simulink model "r4_pfb_fir"  (Simulink 7.0)
settings: Solver=FixedStepDiscrete  SolverMode=SingleTasking  StartTime=0.0  StopTime=10.0  RelTol=1e-3
undefined symbols (not defined in the file): pfb_coefs
libraries: xbsIndex_r4 x385, xps_library x1
(part 13 of 27)

== system r4_pfb_fir/fir_1/fir_tap_2/fir_coef ==
  data_in : Inport  OutDataType=sfix(16)  OutScaling=2^0
  sum_in : Inport  Port=2  OutDataType=sfix(16)  OutScaling=2^0
  sync_in : Inport  Port=3  OutDataType=sfix(16)  OutScaling=2^0
  c_gen : Subsystem  mask(Coefficient Generator){coefs=[-0.000375660323525046;-0.00112528207646786;-0.00187263770065757;-0.00261772609063303;-0.00336054616203061;-0.00410109685156988;-0.00483937711704019;-0.00557538593728603;-0.00630912231219222;-0.00704058526266978;-0.00776977383064064;-0.00849668707902262;-0.00922132409171369;-0.00994368397357705;-0.0106637658504249;-0.0113815688690025;-0.0120970921969721;-0.0128103350228962;-0.0135212965562215;-0.0142299760272615;-0.0149363726871797;-0.0156404858079725;-0.0163423146824514;-0.0170418586242254;-0.0177391169676835;-0.0184340890679761;-0.0191267743009973;-0.0198171720633655;-0.0205052817724058;-0.0211911028661302;-0.0218746348032188;-0.0225558770630009;-0.0232348291454347;-0.0239114905710882;-0.0245858608811188;-0.0252579396372536;-0.0259277264217688;-0.0265952208374693;-0.0272604225076676;-0.0279233310761635;-0.0285839462072226;-0.0292422675855545;-0.0298982949162921;-0.0305520279249694;-0.0312034663574997;-0.031852609980153;-0.0324994585795345;-0.0331440119625613;-0.0337862699564402;-0.0344262324086442;-0.0350638991868898;-0.0356992701791137;-0.0363323452934489;-0.0369631244582015;-0.0375916076218262;-0.0382177947529027;-0.0388416858401109;-0.0394632808922069;-0.0400825799379981;-0.0406995830263182;-0.0413142902260021;-0.0419267016258609;-0.0425368173346564;-0.0431446374810749;-0.0437501622137022;-0.0443533917009969;-0.0449543261312647;-0.0455529657126312;-0.0461493106730163;-0.0467433612601067;-0.047335117741329;-0.0479245804038229;-0.0485117495544134;-0.0490966255195838;-0.0496792086454471;-0.0502594992977191;-0.0508374978616896;-0.0514132047421944;-0.0519866203635867;-0.0525577451697087;-0.0531265796238626;-0.0536931242087811;-0.0542573794265993;-0.0548193457988244;-0.0553790238663066;-0.0559364141892089;-0.0564915173469777;-0.0570443339383125;-0.0575948645811356;-0.0581431099125613;-0.058689070588866;-0.0592327472854569;-0.0597741406968409;-0.0603132515365938;-0.0608500805373288;-0.0613846284506648;-0.0619168960471949;-0.0624468841164546;-0.0629745934668896;-0.0635000249258237;-0.064023179339426;-0.0645440575726791;-0.0650626605093458;-0.0655789890519362;-0.0660930441216749;-0.0666048266584676;-0.0671143376208679;-0.067621577986043;-0.0681265487497408;-0.0686292509262558;-0.0691296855483946;-0.0696278536674418;-0.0701237563531258;-0.0706173946935843;-0.071108769795329;-0.071597882783211;-0.0720847348003859;-0.0725693270082785;-0.0730516605865468;-0.0735317367330474;-0.0740095566637989;-0.0744851216129466;-0.0749584328327259;-0.0754294915934268;-0.0758982991833568;-0.0763648569088048;-0.0768291660940042;-0.0772912280810962;-0.0777510442300928;-0.0782086159188393;-0.0786639445429775;-0.0791170315159078;-0.0795678782687517;-0.0800164862503141;-0.0804628569270452;-0.0809069917830028;-0.0813488923198131;-0.0817885600566336;-0.0822259965301136;-0.0826612032943558;-0.0830941819208773;-0.0835249339985711;-0.0839534611336661;-0.0843797649496887;-0.0848038470874227;-0.0852257092048699;-0.0856453529772106;-0.0860627800967632;-0.0864779922729447;-0.0868909912322302;-0.0873017787181127;-0.0877103564910625;-0.0881167263284868;-0.0885208900246886;-0.0889228493908263;-0.0893226062548723;-0.0897201624615717;-0.0901155198724016;-0.0905086803655288;-0.0908996458357691;-0.0912884181945446;-0.0916749993698427;-0.0920593913061736;-0.0924415959645284;-0.0928216153223364;-0.0931994513734234;-0.0935751061279683;-0.0939485816124612;-0.09431987986966;-0.0946890029585477;-0.0950559529542894;-0.0954207319481889;-0.0957833420476455;-0.0961437853761105;-0.0965020640730433;-0.0968581802938682;-0.0972121362099301;-0.0975639340084509;-0.0979135758924848;-0.0982610640808748;-0.0986064008082076;-0.0989495883247697;-0.0992906288965024;-0.0996295248049575;-0.0999662783472516;-0.100300891836022;-0.100633367599381;-0.100963707980872;-0.101291915339421;-0.101617992049296;-0.101941940500055;-0.102263763096507;-0.102583462258662;-0.102901040421687;-0.103216500035856;-0.103529843566511;-0.103841073494009;-0.104150192313679;-0.104457202535775;-0.104762106685429 ...(+16057 chars)], n_bits=9, bin_pt=8, log2_cpc=0, use_bram=on}
      mask prompts: coefs "Coefficients"; n_bits "Number of Bits"; bin_pt "Binary Point"; log2_cpc "Log2 Cycles per Coefficient"; use_bram "Use BRAM"
      mask help: A coefficient generator.
      settings: AttributesFormatString=|
      | 1024 coefs in bram
      | 9_8 out/1
      mask Help:
      | <pre>
      | Description::
      | 
      | A coefficient generator.
      | 
      | Mask Parameters::
      | 
      | Coefficiants (coefs): The coefficients to output.  These should be specified as doubles.
      | They will be rounded/saturated according to the specified number of bits (n_bits)
      | and binary point (bin_pt).
      | 
      | Number of Coefficient Bits (n_bits): The number of bits used for the fixed point binary
      | representation of the coefficients.
      | 
      | Coefficient Binary Point (bin_pt): The binary point of the fixed point binary representation
      | of the coefficients.
      | 
      | Log2 Cycles per Coefficient (log2_cpc): The log2 value of the number of cycles per coefficient.
      | Must be a non-negative integer (i.e. cycles per coefficient must be a power of 2).
      | 
      | Use BRAM (use_bram): Check this checkbox to store coefficients in BRAM.
      | If unchecked, the coefficients will be sored in distributed memory (i.e. slices).
      | </pre>
  data_delay : xbsIndex_r4/Delay  en=off  latency=1  dbl_ovrd=off  reg_retiming=off  block_type=delay
      settings: xl_area=[0, 0, 0, 0, 0, 0, 0]
  sum_delay : xbsIndex_r4/Delay  en=off  latency=1  dbl_ovrd=off  reg_retiming=off  block_type=delay
      settings: xl_area=[0, 0, 0, 0, 0, 0, 0]
  sync_delay : xbsIndex_r4/Delay  en=off  latency=1  dbl_ovrd=off  reg_retiming=off  block_type=delay
      settings: xl_area=[0, 0, 0, 0, 0, 0, 0]
  data_out : Outport  OutDataType=sfix(16)  OutScaling=2^0
  sum_out : Outport  Port=2  OutDataType=sfix(16)  OutScaling=2^0
  coef : Outport  Port=3  OutDataType=sfix(16)  OutScaling=2^0
  sync_out : Outport  Port=4  OutDataType=sfix(16)  OutScaling=2^0
  wires:
  c_gen/1(coef_out) -> coef/1
  sum_delay/1 -> sum_out/1
  sum_in/1 -> sum_delay/1
  sync_in/1 -> c_gen/1(sync_in), sync_delay/1
  sync_delay/1 -> sync_out/1
  data_delay/1 -> data_out/1
  data_in/1 -> data_delay/1

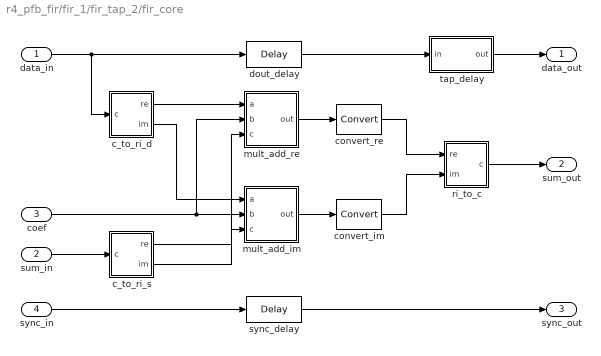
== system r4_pfb_fir/fir_1/fir_tap_2/fir_core ==
  data_in : Inport  OutDataType=sfix(16)  OutScaling=2^0
  sum_in : Inport  Port=2  OutDataType=sfix(16)  OutScaling=2^0
  coef : Inport  Port=3  OutDataType=sfix(16)  OutScaling=2^0
  sync_in : Inport  Port=4  OutDataType=sfix(16)  OutScaling=2^0
  c_to_ri_d : Subsystem  mask(Complex to Real-Imag){n_bits=8, bin_pt=7}
      mask prompts: n_bits "Bit Width"; bin_pt "Binary Point"
      mask help: Outputs real and imaginary components of a complex input.
      settings: AttributesFormatString=8_7 r/i
      mask Help:
      | <pre>
      | Description::
      | 
      | Outputs real and imaginary components of a complex input.
      | Useful for simplifying interconnects.
      | See also: Real-Imag to Complex (ri_to_c)
      | 
      | Mask Parameters::
      | 
      | Bit Width (n_bits): Specifies the width of the real/imaginary components.
      | Assumed equal for both components.
      | 
      | Binary Point (bin_pt): Specifies the binary point location in the real/imaginary components.
      | Assumed equal for both components.
      | </pre>
  c_to_ri_s : Subsystem  mask(Complex to Real-Imag){n_bits=17, bin_pt=15}
      mask prompts: n_bits "Bit Width"; bin_pt "Binary Point"
      mask help: Outputs real and imaginary components of a complex input.
      settings: AttributesFormatString=17_15 r/i
      mask Help:
      | <pre>
      | Description::
      | 
      | Outputs real and imaginary components of a complex input.
      | Useful for simplifying interconnects.
      | See also: Real-Imag to Complex (ri_to_c)
      | 
      | Mask Parameters::
      | 
      | Bit Width (n_bits): Specifies the width of the real/imaginary components.
      | Assumed equal for both components.
      | 
      | Binary Point (bin_pt): Specifies the binary point location in the real/imaginary components.
      | Assumed equal for both components.
      | </pre>
  convert_im : xbsIndex_r4/Convert  arith_type="Signed  (2's comp)"  n_bits=17  bin_pt=15  quantization=Truncate  overflow=Wrap  latency=0  dbl_ovrd=off  pipeline=on  block_type=convert
      settings: xl_area=[0, 0, 0, 0, 0, 0, 0]  block_version=10.1.3
  convert_re : xbsIndex_r4/Convert  arith_type="Signed  (2's comp)"  n_bits=17  bin_pt=15  quantization=Truncate  overflow=Wrap  latency=0  dbl_ovrd=off  pipeline=on  block_type=convert
      settings: xl_area=[0, 0, 0, 0, 0, 0, 0]  block_version=10.1.3
  dout_delay : xbsIndex_r4/Delay  en=off  latency=4  dbl_ovrd=off  reg_retiming=off  block_type=delay
      settings: xl_area=[0, 0, 0, 0, 0, 0, 0]
  mult_add_im : Subsystem  mask(Multiply Add Block){mult_latency=3, add_latency=1, add_bypass=off}
      mask prompts: mult_latency "Multiplier Latency"; add_latency "Adder Latency"; add_bypass "Bypass Adder"
      mask help: A full precision multiply-add block. Produces a*b+c at its ab_c output. The add operation can be optionally bypassed.
      settings: AttributesFormatString=|
      | out = a*b+c
      | latency = 4
      mask Help:
      | <pre>
      | Description::
      | 
      | This full precision multiply-add block produces a*b+c at its ab_c output.
      | The add operation can be optionally bypassed.
      | 
      | Latency is one multiplier latency plus one adder latency (if not bypassing adder).
      | 
      | Mask Parameters::
      | 
      | Multiplier Latency (mult_latency): Latency to use for the underlying real multipliers.
      | 
      | Adder Latency (add_latency): Latency to use for the underlying real adders.
      | 
      | Bypass Adder (add_bypass): Check this checkbox to bypass the adder.
      | </pre>
  mult_add_re : Subsystem  mask(Multiply Add Block){mult_latency=3, add_latency=1, add_bypass=off}
      mask prompts: mult_latency "Multiplier Latency"; add_latency "Adder Latency"; add_bypass "Bypass Adder"
      mask help: A full precision multiply-add block. Produces a*b+c at its ab_c output. The add operation can be optionally bypassed.
      settings: AttributesFormatString=|
      | out = a*b+c
      | latency = 4
      mask Help:
      | <pre>
      | Description::
      | 
      | This full precision multiply-add block produces a*b+c at its ab_c output.
      | The add operation can be optionally bypassed.
      | 
      | Latency is one multiplier latency plus one adder latency (if not bypassing adder).
      | 
      | Mask Parameters::
      | 
      | Multiplier Latency (mult_latency): Latency to use for the underlying real multipliers.
      | 
      | Adder Latency (add_latency): Latency to use for the underlying real adders.
      | 
      | Bypass Adder (add_bypass): Check this checkbox to bypass the adder.
      | </pre>
  ri_to_c : Subsystem  mask(Real-Imag to Complex){}
      mask help: Concatenates real and imaginary inputs into a complex output.
      mask init:
      | ri_to_c_init(gcb);
      mask Help:
      | <pre>
      | Description::
      | 
      | Concatenates a real and imaginary input into a complex output.
      | Useful for simplifying interconnects.
      | See also: Complex to Real-Imag (c_to_ri)
      | 
      | Mask Parameters::
      | 
      | (N/A)
      | </pre>
  sync_delay : xbsIndex_r4/Delay  en=off  latency=4  dbl_ovrd=off  reg_retiming=off  block_type=delay
      settings: xl_area=[0, 0, 0, 0, 0, 0, 0]
  tap_delay : Subsystem  mask(BRAM Delay){delay_depth=1024, buffer_latency=}
      mask prompts: delay_depth "Delay Depth"; buffer_latency "Buffer Latency"
      mask help: A delay block that uses BRAM for its storage.
      settings: AttributesFormatString=bram depth = 1024
      mask Help:
      | <pre>
      | Description::
      | 
      | A delay block that uses BRAM for its storage.
      | 
      | Mask Parameters::
      | 
      | Delay Depth (delay_depth): The length of the delay.
      | 
      | Buffer Latency (buffer_latency): The latency of the underlying storage.
      | 
      | Buffer Latency defaults to 1 and cannot be changed via the block's dialog box.
      | Future versions may enable the setting of that parameter from the dialog.
      | </pre>
  data_out : Outport  OutDataType=sfix(16)  OutScaling=2^0
  sum_out : Outport  Port=2  OutDataType=sfix(16)  OutScaling=2^0
  sync_out : Outport  Port=3  OutDataType=sfix(16)  OutScaling=2^0
  wires:
  convert_im/1 -> ri_to_c/2(im)
  convert_re/1 -> ri_to_c/1(re)
  tap_delay/1(out) -> data_out/1
  mult_add_im/1(out) -> convert_im/1
  mult_add_re/1(out) -> convert_re/1
  c_to_ri_s/2(im) -> mult_add_im/3(c)
  c_to_ri_s/1(re) -> mult_add_re/3(c)
  sum_in/1 -> c_to_ri_s/1(c)
  coef/1 -> mult_add_re/2(b), mult_add_im/2(b)
  c_to_ri_d/2(im) -> mult_add_im/1(a)
  c_to_ri_d/1(re) -> mult_add_re/1(a)
  data_in/1 -> c_to_ri_d/1(c), dout_delay/1
  dout_delay/1 -> tap_delay/1(in)
  ri_to_c/1(c) -> sum_out/1
  sync_delay/1 -> sync_out/1
  sync_in/1 -> sync_delay/1
